simulink model "differential_equations"  (R2017b)
settings: Solver=VariableStepAuto  StartTime=0.0  StopTime=10.0  RelTol=1e-3
values from neighbouring files (symbols this model uses):
  k1 = 2    [differential_equations_parameters.m]
  k2 = 2    [differential_equations_parameters.m]
  k3 = 2    [differential_equations_parameters.m]
  m1 = 2    [differential_equations_parameters.m]
  m2 = 3    [differential_equations_parameters.m]
  m4 = 7    [differential_equations_parameters.m]
settings Model: Creator=Damla  LastModifiedBy=dagac

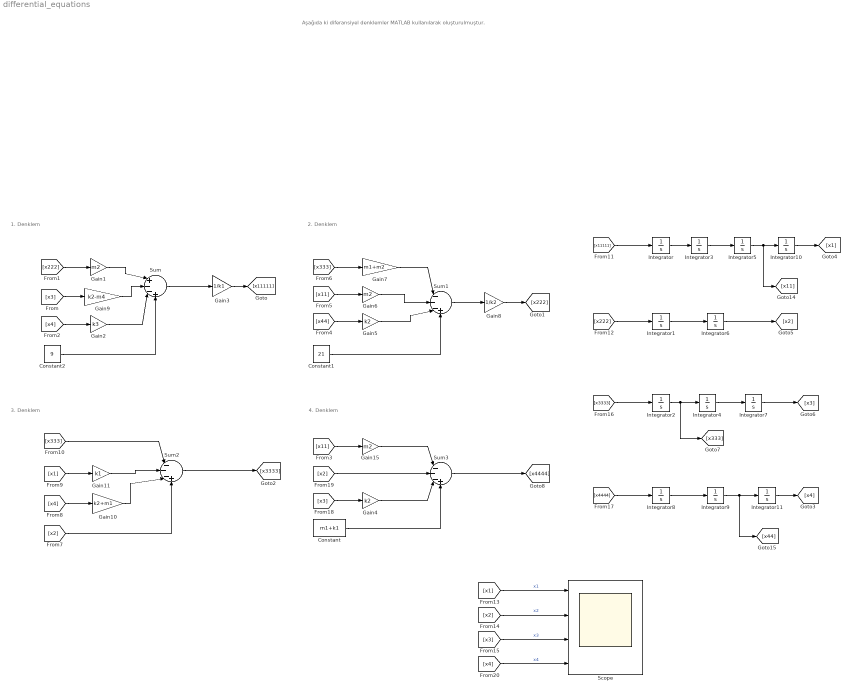
== system differential_equations ==
  note: Aşağıda ki diferansiyel denklemler MATLAB kullanılarak oluşturulmuştur.
  note: 1. Denklem
  note: 2. Denklem
  note: 4. Denklem
  note: 3. Denklem
  Constant : Constant  Value=m1+k1
  Constant1 : Constant  Value=21
  Constant2 : Constant  Value=9
  Gain1 : Gain  Gain=m2
  Gain10 : Gain  Gain=k2+m1
  Gain11 : Gain  Gain=k1
  Gain15 : Gain  Gain=m2
  Gain2 : Gain  Gain=k3
  Gain3 : Gain  Gain=1/k1
  Gain4 : Gain  Gain=k2
  Gain5 : Gain  Gain=k2
  Gain6 : Gain  Gain=m2
  Gain7 : Gain  Gain=m1+m2
  Gain8 : Gain  Gain=1/k2
  Gain9 : Gain  Gain=k2-m4
  Integrator{,1..11} (12 alike) : Integrator
  Scope : Scope  NumInputPorts=4
  Sum : Sum  Inputs=|+--+
  Sum1 : Sum  Inputs=|---+
  Sum2 : Sum  Inputs=|---+
  Sum3 : Sum  Inputs=|---+
  wires:
  Gain2/1 -> Sum/3
  [x222] -> Integrator1/1
  [x3333] -> Integrator2/1
  Gain5/1 -> Sum1/3
  [x4] -> Gain10/1
  [x2] -> Sum2/4
  Integrator7/1 -> [x3]
  Gain4/1 -> Sum3/3
  Constant/1 -> Sum3/4
  Constant2/1 -> Sum/4
  Gain8/1 -> [x222]
  Sum1/1 -> Gain8/1
  [x2] -> Sum3/2
  [x11] -> Gain15/1
  [x4444] -> Integrator8/1
  Gain11/1 -> Sum2/2
  Integrator3/1 -> Integrator5/1
  Integrator9/1 -> [x44], Integrator11/1
  [x44] -> Gain5/1
  Gain7/1 -> Sum1/1
  [x3] -> Gain4/1
  Integrator5/1 -> [x11], Integrator10/1
  Gain6/1 -> Sum1/2
  Sum3/1 -> [x4444]
  Integrator8/1 -> Integrator9/1
  Constant1/1 -> Sum1/4
  [x333] -> Sum2/1
  Integrator/1 -> Integrator3/1
  Integrator4/1 -> Integrator7/1
  Integrator6/1 -> [x2]
  Gain3/1 -> [x11111]
  Integrator2/1 -> [x333], Integrator4/1
  [x4] -> Gain2/1
  Gain15/1 -> Sum3/1
  [x3] -> Gain9/1
  [x11111] -> Integrator/1
  [x222] -> Gain1/1
  [x11] -> Gain6/1
  [x1] -> Gain11/1
  Sum2/1 -> [x3333]
  Sum/1 -> Gain3/1
  [x333] -> Gain7/1
  Integrator1/1 -> Integrator6/1
  Gain10/1 -> Sum2/3
  Gain1/1 -> Sum/1
  Gain9/1 -> Sum/2
  Integrator10/1 -> [x1]
  Integrator11/1 -> [x4]
  [x2] -> Scope/2  "x2"
  [x1] -> Scope/1  "x1"
  [x3] -> Scope/3  "x3"
  [x4] -> Scope/4  "x4"
